simulink model "assignment_2_simulink_q6"  (R2023a)
settings: Solver=VariableStepAuto  StartTime=0.0  StopTime=10.0  RelTol=1e-3
undefined symbols (not defined in the file or in its folder): ki, kp, kt
settings Model: Creator=chowd  LastModifiedBy=chowd

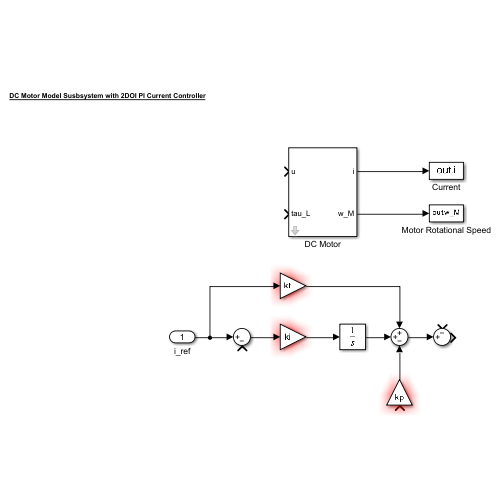
[thumbnail: Simulink's stored preview of the top-level diagram]
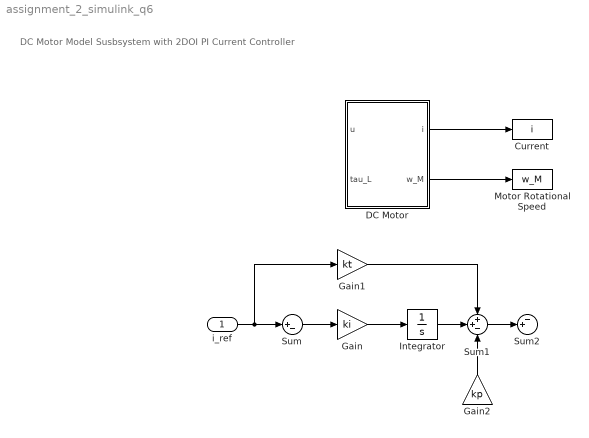
== system assignment_2_simulink_q6 ==
  note: DC Motor Model Susbsystem with 2DOI PI Current Controller
  i_ref : Inport
  Current : ToWorkspace  VariableName=i  SaveFormat=Timeseries  SampleTime=-1
  DC Motor : Subsystem  mask{R=0.5, L=2.5e-3, k=0.35, J=1e-3}
      mask prompts: R "R (ohm)"; L "L (H)"; k "k (Vs)"; J "J (kgm^2)"
  Gain : Gain  Gain=ki
  Gain1 : Gain  Gain=kt
  Gain2 : Gain  Gain=kp
  Integrator : Integrator
  Motor Rotational Speed : ToWorkspace  VariableName=w_M  SaveFormat=Timeseries  SampleTime=-1
  Sum : Sum  Inputs=|+-
  Sum1 : Sum  Inputs=++-
  Sum2 : Sum  Inputs=-+|
  wires:
  DC Motor/1(i) -> Current/1
  DC Motor/2(w_M) -> Motor Rotational Speed/1
  i_ref/1 -> Gain1/1, Sum/1
  Sum/1 -> Gain/1
  Gain/1 -> Integrator/1
  Integrator/1 -> Sum1/2
  Sum1/1 -> Sum2/2
  Gain1/1 -> Sum1/1
  Gain2/1 -> Sum1/3

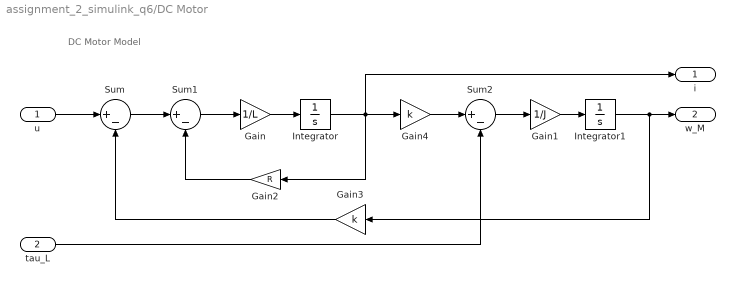
== system assignment_2_simulink_q6/DC Motor ==
  note: DC Motor Model
  u : Inport
  tau_L : Inport  Port=2
  Gain : Gain  Gain=1/L
  Gain1 : Gain  Gain=1/J
  Gain2 : Gain  Gain=R
  Gain3 : Gain  Gain=k
  Gain4 : Gain  Gain=k
  Integrator : Integrator
  Integrator1 : Integrator
  Sum : Sum  Inputs=|+-
  Sum1 : Sum  Inputs=|+-
  Sum2 : Sum  Inputs=|+-
  i : Outport
  w_M : Outport  Port=2
  wires:
  Gain/1 -> Integrator/1
  Sum2/1 -> Gain1/1
  Sum/1 -> Sum1/1
  u/1 -> Sum/1
  Integrator/1 -> Gain2/1, i/1, Gain4/1
  Sum1/1 -> Gain/1
  Gain2/1 -> Sum1/2
  Gain3/1 -> Sum/2
  tau_L/1 -> Sum2/2
  Integrator1/1 -> w_M/1, Gain3/1
  Gain4/1 -> Sum2/1
  Gain1/1 -> Integrator1/1
